simulink model "Tires"  (R2023a)
settings: Solver=VariableStepAuto  StartTime=0.0  StopTime=10.0  RelTol=1e-3
undefined symbols (not defined in the file): C, C_alpha_f, C_r, E, e_p0, g, l_f, l_r, m, n_st
settings Model: Creator=Tan_Tram  LastModifiedBy=Tan_Tram

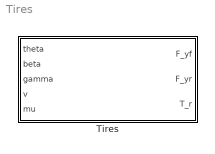
== system Tires ==
  Tires : Subsystem

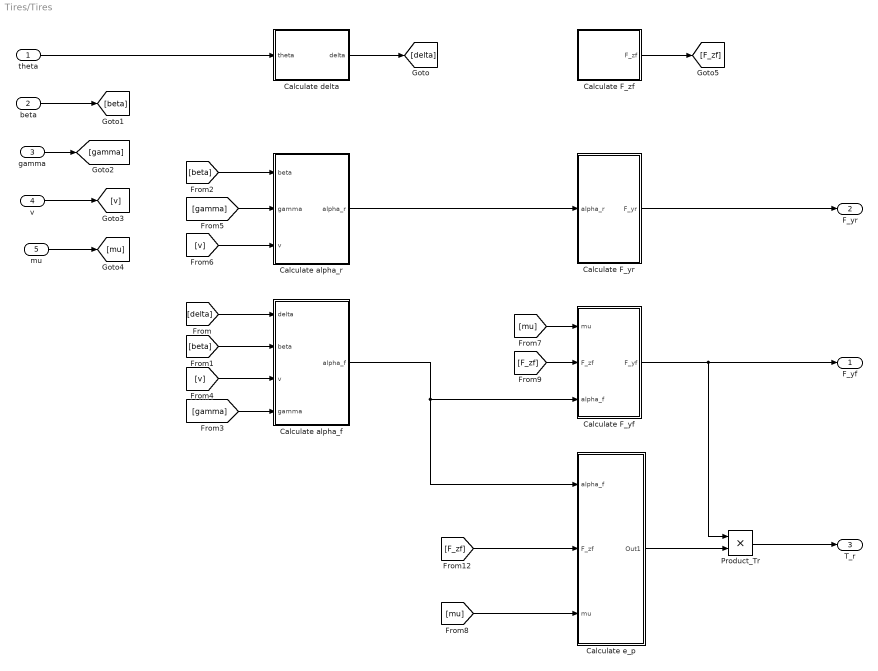
== system Tires/Tires ==
  theta : Inport
  beta : Inport  Port=2
  gamma : Inport  Port=3
  v : Inport  Port=4
  mu : Inport  Port=5
  Calculate F_yf : Subsystem
  Calculate F_yr : Subsystem
  Calculate F_zf : Subsystem
  Calculate alpha_f : Subsystem
  Calculate alpha_r : Subsystem
  Calculate delta : Subsystem
  Calculate e_p : Subsystem
  Product_Tr : Product  Inputs=**
  F_yf : Outport
  F_yr : Outport  Port=2
  T_r : Outport  Port=3
  wires:
  Product_Tr/1 -> T_r/1
  theta/1 -> Calculate delta/1(theta)
  [delta] -> Calculate alpha_f/1(delta)
  Calculate delta/1(delta) -> [delta]
  beta/1 -> [beta]
  [beta] -> Calculate alpha_f/2(beta)
  gamma/1 -> [gamma]
  [gamma] -> Calculate alpha_f/4(gamma)
  v/1 -> [v]
  [v] -> Calculate alpha_f/3(v)
  [beta] -> Calculate alpha_r/1(beta)
  [gamma] -> Calculate alpha_r/2(gamma)
  [v] -> Calculate alpha_r/3(v)
  mu/1 -> [mu]
  Calculate F_zf/1(F_zf) -> [F_zf]
  Calculate F_yf/1(F_yf) -> F_yf/1, Product_Tr/1
  [mu] -> Calculate F_yf/1(mu)
  [F_zf] -> Calculate F_yf/2(F_zf)
  Calculate alpha_r/1(alpha_r) -> Calculate F_yr/1(alpha_r)
  Calculate F_yr/1(F_yr) -> F_yr/1
  Calculate alpha_f/1(alpha_f) -> Calculate F_yf/3(alpha_f), Calculate e_p/1(alpha_f)
  [F_zf] -> Calculate e_p/2(F_zf)
  [mu] -> Calculate e_p/3(mu)
  Calculate e_p/1(Out1) -> Product_Tr/2

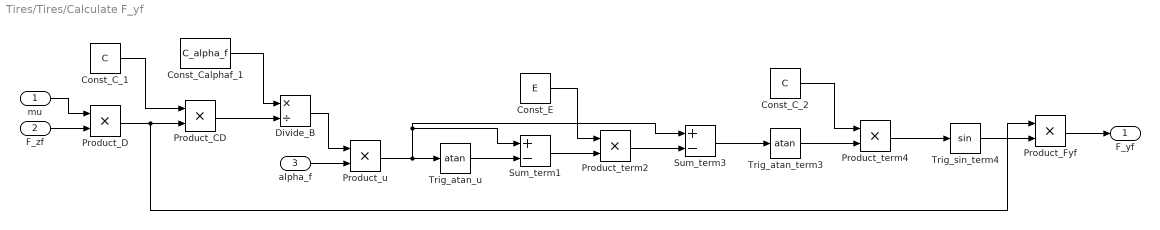
== system Tires/Tires/Calculate F_yf ==
  mu : Inport
  F_zf : Inport  Port=2
  alpha_f : Inport  Port=3
  Const_C_1 : Constant  Value=C
  Const_C_2 : Constant  Value=C
  Const_Calphaf_1 : Constant  Value=C_alpha_f
  Const_E : Constant  Value=E
  Divide_B : Product  Inputs=*/
  Product_CD : Product  Inputs=**
  Product_D : Product  Inputs=**
  Product_Fyf : Product  Inputs=**
  Product_term2 : Product  Inputs=**
  Product_term4 : Product  Inputs=**
  Product_u : Product  Inputs=**
  Sum_term1 : Sum  Inputs=+-
  Sum_term3 : Sum  Inputs=+-
  Trig_atan_term3 : Trigonometry  Operator=atan
  Trig_atan_u : Trigonometry  Operator=atan
  Trig_sin_term4 : Trigonometry
  F_yf : Outport
  wires:
  alpha_f/1 -> Product_u/2
  Sum_term1/1 -> Product_term2/2
  Divide_B/1 -> Product_u/1
  F_zf/1 -> Product_D/2
  mu/1 -> Product_D/1
  Const_Calphaf_1/1 -> Divide_B/1
  Const_E/1 -> Product_term2/1
  Const_C_1/1 -> Product_CD/1
  Product_CD/1 -> Divide_B/2
  Product_D/1 -> Product_CD/2, Product_Fyf/1
  Sum_term3/1 -> Trig_atan_term3/1
  Product_u/1 -> Sum_term3/1, Sum_term1/1, Trig_atan_u/1
  Trig_atan_u/1 -> Sum_term1/2
  Product_term2/1 -> Sum_term3/2
  Const_C_2/1 -> Product_term4/1
  Trig_atan_term3/1 -> Product_term4/2
  Product_term4/1 -> Trig_sin_term4/1
  Trig_sin_term4/1 -> Product_Fyf/2
  Product_Fyf/1 -> F_yf/1

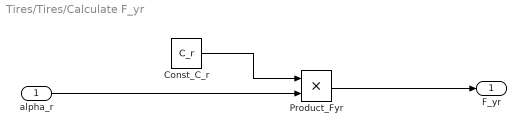
== system Tires/Tires/Calculate F_yr ==
  alpha_r : Inport
  Const_C_r : Constant  Value=C_r
  Product_Fyr : Product  Inputs=**
  F_yr : Outport
  wires:
  Const_C_r/1 -> Product_Fyr/1
  alpha_r/1 -> Product_Fyr/2
  Product_Fyr/1 -> F_yr/1

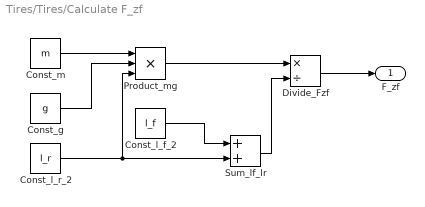
== system Tires/Tires/Calculate F_zf ==
  Const_g : Constant  Value=g
  Const_l_f_2 : Constant  Value=l_f
  Const_l_r_2 : Constant  Value=l_r
  Const_m : Constant  Value=m
  Divide_Fzf : Product  Inputs=*/
  Product_mg : Product  Inputs=***
  Sum_lf_lr : Sum
  F_zf : Outport
  wires:
  Const_l_r_2/1 -> Sum_lf_lr/2, Product_mg/3
  Divide_Fzf/1 -> F_zf/1
  Product_mg/1 -> Divide_Fzf/1
  Const_m/1 -> Product_mg/1
  Const_g/1 -> Product_mg/2
  Sum_lf_lr/1 -> Divide_Fzf/2
  Const_l_f_2/1 -> Sum_lf_lr/1

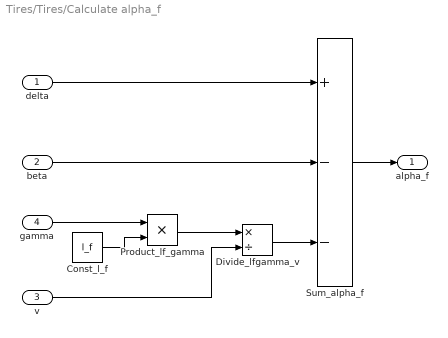
== system Tires/Tires/Calculate alpha_f ==
  delta : Inport
  beta : Inport  Port=2
  v : Inport  Port=3
  gamma : Inport  Port=4
  Const_l_f : Constant  Value=l_f
  Divide_lfgamma_v : Product  Inputs=*/
  Product_lf_gamma : Product  Inputs=**
  Sum_alpha_f : Sum  Inputs=+--
  alpha_f : Outport
  wires:
  delta/1 -> Sum_alpha_f/1
  beta/1 -> Sum_alpha_f/2
  v/1 -> Divide_lfgamma_v/2
  gamma/1 -> Product_lf_gamma/1
  Product_lf_gamma/1 -> Divide_lfgamma_v/1
  Divide_lfgamma_v/1 -> Sum_alpha_f/3
  Sum_alpha_f/1 -> alpha_f/1
  Const_l_f/1 -> Product_lf_gamma/2

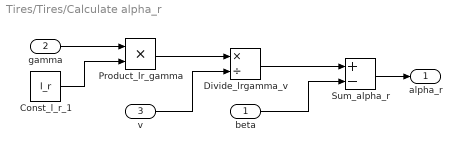
== system Tires/Tires/Calculate alpha_r ==
  beta : Inport
  gamma : Inport  Port=2
  v : Inport  Port=3
  Const_l_r_1 : Constant  Value=l_r
  Divide_lrgamma_v : Product  Inputs=*/
  Product_lr_gamma : Product  Inputs=**
  Sum_alpha_r : Sum  Inputs=+-
  alpha_r : Outport
  wires:
  gamma/1 -> Product_lr_gamma/1
  Const_l_r_1/1 -> Product_lr_gamma/2
  Product_lr_gamma/1 -> Divide_lrgamma_v/1
  v/1 -> Divide_lrgamma_v/2
  Sum_alpha_r/1 -> alpha_r/1
  beta/1 -> Sum_alpha_r/2
  Divide_lrgamma_v/1 -> Sum_alpha_r/1

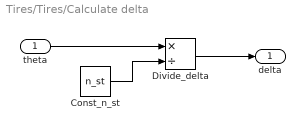
== system Tires/Tires/Calculate delta ==
  theta : Inport
  Const_n_st : Constant  Value=n_st
  Divide_delta : Product  Inputs=*/
  delta : Outport
  wires:
  theta/1 -> Divide_delta/1
  Divide_delta/1 -> delta/1
  Const_n_st/1 -> Divide_delta/2

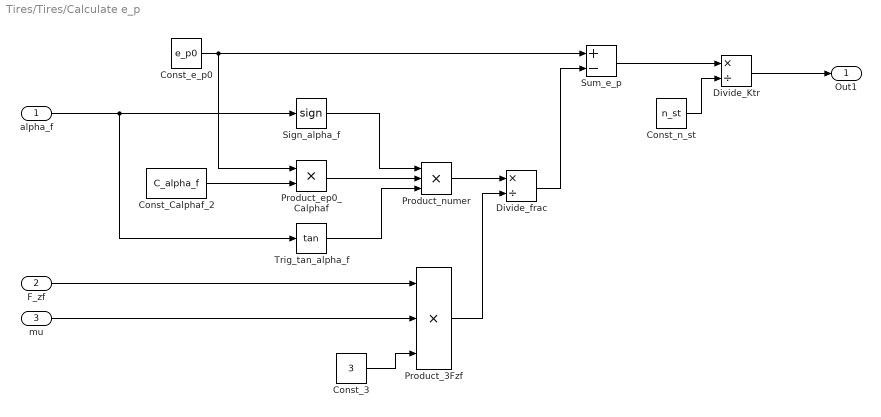
== system Tires/Tires/Calculate e_p ==
  alpha_f : Inport
  F_zf : Inport  Port=2
  mu : Inport  Port=3
  Const_3 : Constant  Value=3
  Const_Calphaf_2 : Constant  Value=C_alpha_f
  Const_e_p0 : Constant  Value=e_p0
  Const_n_st : Constant  Value=n_st
  Divide_Ktr : Product  Inputs=*/
  Divide_frac : Product  Inputs=*/
  Product_3Fzf : Product  Inputs=***
  Product_ep0_Calphaf : Product  Inputs=**
  Product_numer : Product  Inputs=***
  Sign_alpha_f : Signum
  Sum_e_p : Sum  Inputs=+-
  Trig_tan_alpha_f : Trigonometry  Operator=tan
  Out1 : Outport
  wires:
  Sum_e_p/1 -> Divide_Ktr/1
  Trig_tan_alpha_f/1 -> Product_numer/3
  alpha_f/1 -> Trig_tan_alpha_f/1, Sign_alpha_f/1
  Sign_alpha_f/1 -> Product_numer/1
  Product_ep0_Calphaf/1 -> Product_numer/2
  Product_numer/1 -> Divide_frac/1
  Const_e_p0/1 -> Sum_e_p/1, Product_ep0_Calphaf/1
  mu/1 -> Product_3Fzf/2
  Divide_frac/1 -> Sum_e_p/2
  Const_Calphaf_2/1 -> Product_ep0_Calphaf/2
  Const_n_st/1 -> Divide_Ktr/2
  Const_3/1 -> Product_3Fzf/3
  Product_3Fzf/1 -> Divide_frac/2
  Divide_Ktr/1 -> Out1/1
  F_zf/1 -> Product_3Fzf/1
